simulink model "task_3_sim"  (R2023a)
settings: Solver=VariableStepAuto  StartTime=0.0  StopTime=2  MaxStep=1e-5  RelTol=1e-5
undefined symbols (not defined in the file): A, B, K, x0
settings Model: Creator=user  LastModifiedBy=user

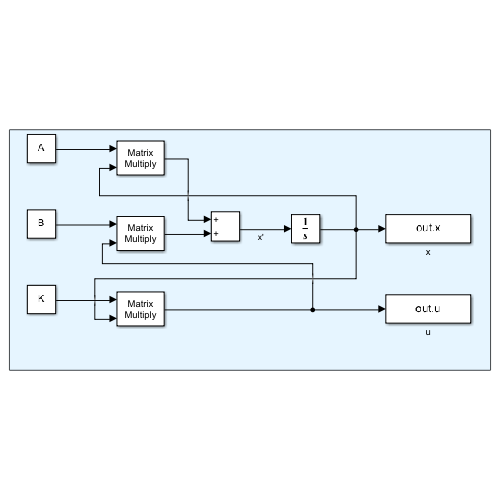
[thumbnail: Simulink's stored preview of the top-level diagram]
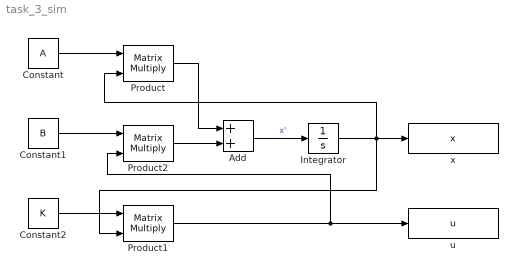
== system task_3_sim ==
  Add : Sum
  Constant : Constant  Value=A
  Constant1 : Constant  Value=B  VectorParams1D=off
  Constant2 : Constant  Value=K  VectorParams1D=off
  Integrator : Integrator  InitialCondition=x0
  Product : Product  Multiplication=Matrix(*)
  Product1 : Product  Multiplication=Matrix(*)
  Product2 : Product  Multiplication=Matrix(*)
  u : ToWorkspace  VariableName=u  SaveFormat=Timeseries  SampleTime=-1
  x : ToWorkspace  VariableName=x  SaveFormat=Timeseries  SampleTime=-1
  wires:
  Integrator/1 -> Product/2, x/1, Product1/2
  Constant2/1 -> Product1/1
  Product2/1 -> Add/2
  Constant/1 -> Product/1
  Add/1 -> Integrator/1  "x'"
  Constant1/1 -> Product2/1
  Product1/1 -> u/1, Product2/2
  Product/1 -> Add/1
